simulink model "PV_UPQC_Final1_MAF_2018a (1)"  (R2018a)
settings: Solver=ode23tb  StartTime=0.0  StopTime=6  FixedStep=Ts_Power  RelTol=1e-4
PreLoadFcn:
  | Ts_Power=50e-6;
  | Ts_Control=100e-6;
InitFcn:
  | Ts_Power=50e-6;
  | Ts_Control=100e-6;
model workspace (MAT data in the model file):
  A = [0  0  0; -1  -1.5  -0.75; 0  1  0]
  B = [0.5; 0; 0]
  C = [0 -1.5 0]
  D = 0
  G = ss
  G.IOSize_ = [1 1]
  G.Data_ = ltipack.ssdata
  G.Data_.a = 0
  G.Data_.b = [0.5 0]
  G.Data_.c = [0.5; -0.5]
  G.Data_.d = [0  1; 0  0]
  G.Data_.Delay.Input = 0
  G.Data_.Delay.Output = 0
  G.Data_.Delay.Internal = 4
  G.Data_.Ts = 0
  Ga = ss
  Ga.IOSize_ = [1 1]
  Ga.Data_ = ltipack.ssdata
  Ga.Data_.a = [0  0  0; -1  -1.5  -0.75; 0  1  0]
  Ga.Data_.b = [0.5; 0; 0]
  Ga.Data_.c = [0 -1.5 0]
  Ga.Data_.d = 0
  Ga.Data_.Delay.Input = 0
  Ga.Data_.Delay.Output = 0
  Ga.Data_.Delay.Internal = []
  Ga.Data_.Ts = 0
  Gtf = tf
  Gtf.IOSize_ = [1 1]
  Gtf.Data_ = ltipack.tfdata
  Gtf.Data_.num = {[1 1.5 0.75 0]}
  Gtf.Data_.den = {[0 0 0.75 0]}
  Gtf.Data_.Delay.Input = 0
  Gtf.Data_.Delay.Output = 0
  Gtf.Data_.Delay.IO = 0
  Gtf.Data_.Ts = 0
  Ts = 2.5e-05
  s = tf
  s.IOSize_ = [1 1]
  s.Data_ = ltipack.tfdata
  s.Data_.num = {[1 0]}
  s.Data_.den = {[0 1]}
  s.Data_.Delay.Input = 0
  s.Data_.Delay.Output = 0
  s.Data_.Delay.IO = 0
  s.Data_.Ts = 0
libraries: powerlib x38, powerlib_meascontrol x12, simulink x4, dspstat3 x1, re_lib x1
Description:
  | Copyright 2008-2017 The MathWorks, Inc.
settings Model: Creator=MathWorks  LastModifiedBy=LMS Solution
settings SolverCC: SolverJacobianMethodControl=FullAnalytical  ZeroCrossAlgorithm=Adaptive  AlgebraicLoopSolver=LineSearch
settings DataIOCC: LimitDataPoints=on  SaveFormat=Array  SignalLoggingSaveFormat=ModelDataLogs
settings OptimizationCC: ExpressionDepthLimit=2147483647  LifeSpan=inf
settings DebuggingCC: UnderspecifiedInitializationDetection=Classic  MergeDetectMultiDrivingBlocksExec=none  SolverPrmCheckMsg=warning  FcnCallInpInsideContextMsg=warning  StateNameClashWarn=warning  SFUnexpectedBacktrackingDiag=warning  SFNoUnconditionalDefaultTransitionDiag=warning  SFExecutionAtInitializationDiag=none
settings HardwareCC: ProdBitPerPointer=32  ProdBitPerSizeT=32  ProdBitPerPtrDiffT=32  ProdLargestAtomicFloat=None  ProdIntDivRoundTo=Undefined  ProdEndianess=Unspecified  ProdWordSize=32  ProdHWDeviceType=32-bit Generic
settings ModelReferenceCC: PropagateSignalLabelsOutOfModel=off
settings CodeAppCC: StateflowObjectComments=on
settings GRTTargetCC: TargetLangStandard=C89/C90 (ANSI)  CombineOutputUpdateFcns=off  GRTInterface=on
settings ConfigComp: CovMetricSettings=dw  CovHtmlReporting=on  CovSaveCumulativeToWorkspaceVar=on  CovSaveSingleToWorkspaceVar=on  CovExternalEMLEnable=off  CovSFcnEnable=off
settings SimscapeCC: SimscapeNormalizeSystem=off

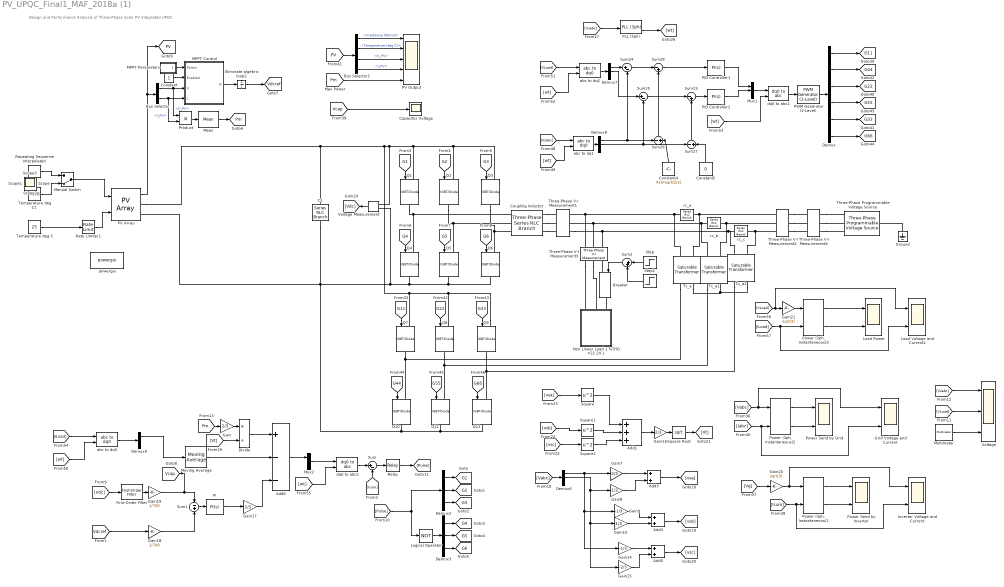
== system PV_UPQC_Final1_MAF_2018a (1) ==
  note: Design and Performance Analysis of Three-Phase Solar PV Integrated UPQC
  Add1 : Sum  Inputs=+++
  Add3 : Sum
  Add4 : Sum
  Add5 : Sum
  Add6 : Sum  Inputs=+--
  Breaker : powerlib/Elements/Breaker  InitialState=0  SwitchingTimes="[1/60  5/60]"  External=on  BreakerResistance=0.01  SnubberResistance=1e6  SnubberCapacitance=inf  Measurements=None  MoreParameters=on  NoBreakLoop=off
  Bus Selector : BusSelector  OutputSignals=V_PV,I_PV
  Bus Selector1 : BusSelector  OutputSignals=Irradiance (W/m2),Temperature (deg C),V_PV,I_PV
  C1 : powerlib/Elements/Series RLC Branch  LConnTagsString=__new0  RConnTagsString=__new0  BranchType=C  Resistance=1  Inductance=1e-3  SetiL0=off  InitialCurrent=0  Capacitance=6668e-6  Setx0=on  InitialVoltage=700  Measurements=None
  Capacitor Voltage : Scope
  Constant : Constant
  Constant4 : Constant  Value=415*sqrt(2/3)
  Constant5 : Constant  Value=0
  Coupling Inductor : powerlib/Elements/Three-Phase Series RLC Branch  LConnTagsString=A|B|C  RConnTagsString=A|B|C  BranchType=L  Resistance=0.09  Inductance=1.39e-3  Capacitance=1e-6  Measurements=None
  Demux : Demux  Outputs=6
  Demux{2..3,6..9} (6 alike) : Demux  Outputs=3
  Divide : Product  Inputs=*/
  Eliminate algebric loop2 : UnitDelay  InitialCondition=0.485  SampleTime=Ts_Control  HasFrameUpgradeWarning=on
  First-Order Filter : powerlib_meascontrol/Filters/First-Order Filter  FilterType=Lowpass  Tc=10e-3  Ts=0  Initialize=on  Vac_Init=[0, 0, 60]  Vdc_Init=0  PlotResponse=off  FreqRange="[0,  200,  1]"
  Gain : Gain  Gain=2/3
  Gain10 : Gain  Gain=1/3
  Gain14 : Gain  Gain=-1/3
  Gain15 : Gain  Gain=-2/3
  Gain16 : Gain  Gain=2/3
  Gain17 : Gain  Gain=1/3
  Gain18 : Gain  Gain=1/700
  Gain19 : Gain  Gain=1/700
  Gain20 : Gain  Gain=sqrt(3)
  Gain21 : Gain  Gain=sqrt(3)
  Gain7 : Gain  Gain=2/3
  Gain8 : Gain  Gain=1/3
  Gain9 : Gain  Gain=-1/3
  Grid Voltage and Current : Scope  NumInputPorts=2
  Ground : powerlib/Elements/Ground  LConnTagsString=a
  Inverter Voltage and Current : Scope  NumInputPorts=2
  Load Power : Scope  NumInputPorts=2
  Load Voltage and Current1 : Scope  NumInputPorts=2
  Logical Operator : Logic  Operator=NOT  IconShape=distinctive  AllPortsSameDT=off  OutDataTypeStr=boolean
  MPPT Parameters : Subsystem
  "MPPT Control  " : MATLAB Function  TreatAsAtomicUnit=on
  Manual Switch : ManualSwitch  CurrentSetting=0
  Mean : powerlib_meascontrol/Measurements/Mean  Freq=50  Vinit=0  Ts=0
  Moving Average : dspstat3/Moving Average  Method=Sliding window  ForgettingFactorPort=off  SpecifyWindowLength=on  WindowLength=4  ForgettingFactor=0.9  SimulateUsing=Code generation
  Multimeter : powerlib/Measurements/Multimeter  PhasorSimulation=off  OutputType=Complex  sel=[1 2 3]  L=3  Gain=[1 1 1]  yselected={'Ub: rc_a','Ub: rc_b','Ub: rc_c'};  PSBOutputType=1  PSBequivalent=0  AxesSetting=[0,0.1,-100,100]  Display=0  SavedBlockNames=-11
  Mux1 : Mux  Inputs=3
  Mux2 : Mux  Inputs=3
  "Non Linear Load { %THD =22.24 }" : Subsystem
      mask Display: fprintf('Non Linear\nLoad')
  PI : simulink/Continuous/PID Controller  Controller=PI  Form=Parallel  TimeDomain=Continuous-time  SampleTime=-1  IntegratorMethod=Forward Euler  FilterMethod=Forward Euler  ControllerParametersSource=internal  P=1000  I=1200  D=0  UseFilter=on  N=100  TunerSelectOption=Transfer Function Based (PID Tuner App)  InitialConditionSource=internal  InitialConditionForIntegrator=0  InitialConditionForFilter=0  DifferentiatorICPrevScaledInput=0  ExternalReset=none  TrackingMode=off  Kt=1  LimitOutput=off  UpperSaturationLimit=inf  LowerSaturationLimit=-inf  LinearizeAsGain=on  AntiWindupMode=none  Kb=1  POutMin=[]  POutMax=[]  IOutMin=[]  IOutMax=[]  DOutMin=[]  DOutMax=[]  NOutMin=[]  NOutMax=[]  SumOutMin=[]  SumOutMax=[]  SaturationOutMin=[]  SaturationOutMax=[]  PParamMin=[]  PParamMax=[]  IParamMin=[]  IParamMax=[]  DParamMin=[]  DParamMax=[]  NParamMin=[]  NParamMax=[]  KbParamMin=[]  KbParamMax=[]  KtParamMin=[]  KtParamMax=[]  KbOutMin=[]  KbOutMax=[]  KtOutMin=[]  KtOutMax=[]  IntegratorOutMin=[]  IntegratorOutMax=[]  FilterOutMin=[]  FilterOutMax=[]  SumI1OutMin=[]  SumI1OutMax=[]  SumI2OutMin=[]  SumI2OutMax=[]  SumI3OutMin=[]  SumI3OutMax=[]  SumDOutMin=[]  SumDOutMax=[]  DifferentiatorOutMin=[]  DifferentiatorOutMax=[]  FilterDiffOutCoefMin=[]  FilterDiffOutCoefMax=[]  ReciprocalOutMin=[]  ReciprocalOutMax=[]  SumDenOutMin=[]  SumDenOutMax=[]  SumNumOutMin=[]  SumNumOutMax=[]  DivideOutMin=[]  DivideOutMax=[]  IntegratorContinuousStateAttributes=''  IntegratorStateMustResolveToSignalObject=off  IntegratorRTWStateStorageClass=Auto  FilterContinuousStateAttributes=''  FilterStateMustResolveToSignalObject=off  FilterRTWStateStorageClass=Auto
  PID Controller1 : simulink/Continuous/PID Controller  Controller=PI  Form=Parallel  TimeDomain=Continuous-time  SampleTime=-1  IntegratorMethod=Forward Euler  FilterMethod=Forward Euler  ControllerParametersSource=internal  P=1  I=1  D=0  UseFilter=on  N=100  TunerSelectOption=Transfer Function Based (PID Tuner App)  InitialConditionSource=internal  InitialConditionForIntegrator=0  InitialConditionForFilter=0  DifferentiatorICPrevScaledInput=0  ExternalReset=none  TrackingMode=off  Kt=1  LimitOutput=off  UpperSaturationLimit=inf  LowerSaturationLimit=-inf  LinearizeAsGain=on  AntiWindupMode=none  Kb=1  POutMin=[]  POutMax=[]  IOutMin=[]  IOutMax=[]  DOutMin=[]  DOutMax=[]  NOutMin=[]  NOutMax=[]  SumOutMin=[]  SumOutMax=[]  SaturationOutMin=[]  SaturationOutMax=[]  PParamMin=[]  PParamMax=[]  IParamMin=[]  IParamMax=[]  DParamMin=[]  DParamMax=[]  NParamMin=[]  NParamMax=[]  KbParamMin=[]  KbParamMax=[]  KtParamMin=[]  KtParamMax=[]  KbOutMin=[]  KbOutMax=[]  KtOutMin=[]  KtOutMax=[]  IntegratorOutMin=[]  IntegratorOutMax=[]  FilterOutMin=[]  FilterOutMax=[]  SumI1OutMin=[]  SumI1OutMax=[]  SumI2OutMin=[]  SumI2OutMax=[]  SumI3OutMin=[]  SumI3OutMax=[]  SumDOutMin=[]  SumDOutMax=[]  DifferentiatorOutMin=[]  DifferentiatorOutMax=[]  FilterDiffOutCoefMin=[]  FilterDiffOutCoefMax=[]  ReciprocalOutMin=[]  ReciprocalOutMax=[]  SumDenOutMin=[]  SumDenOutMax=[]  SumNumOutMin=[]  SumNumOutMax=[]  DivideOutMin=[]  DivideOutMax=[]  IntegratorContinuousStateAttributes=''  IntegratorStateMustResolveToSignalObject=off  IntegratorRTWStateStorageClass=Auto  FilterContinuousStateAttributes=''  FilterStateMustResolveToSignalObject=off  FilterRTWStateStorageClass=Auto
  PID Controller2 : simulink/Continuous/PID Controller  Controller=PI  Form=Parallel  TimeDomain=Continuous-time  SampleTime=-1  IntegratorMethod=Forward Euler  FilterMethod=Forward Euler  ControllerParametersSource=internal  P=8  I=10  D=0  UseFilter=on  N=100  TunerSelectOption=Transfer Function Based (PID Tuner App)  InitialConditionSource=internal  InitialConditionForIntegrator=0  InitialConditionForFilter=0  DifferentiatorICPrevScaledInput=0  ExternalReset=none  TrackingMode=off  Kt=1  LimitOutput=off  UpperSaturationLimit=inf  LowerSaturationLimit=-inf  LinearizeAsGain=on  AntiWindupMode=none  Kb=1  POutMin=[]  POutMax=[]  IOutMin=[]  IOutMax=[]  DOutMin=[]  DOutMax=[]  NOutMin=[]  NOutMax=[]  SumOutMin=[]  SumOutMax=[]  SaturationOutMin=[]  SaturationOutMax=[]  PParamMin=[]  PParamMax=[]  IParamMin=[]  IParamMax=[]  DParamMin=[]  DParamMax=[]  NParamMin=[]  NParamMax=[]  KbParamMin=[]  KbParamMax=[]  KtParamMin=[]  KtParamMax=[]  KbOutMin=[]  KbOutMax=[]  KtOutMin=[]  KtOutMax=[]  IntegratorOutMin=[]  IntegratorOutMax=[]  FilterOutMin=[]  FilterOutMax=[]  SumI1OutMin=[]  SumI1OutMax=[]  SumI2OutMin=[]  SumI2OutMax=[]  SumI3OutMin=[]  SumI3OutMax=[]  SumDOutMin=[]  SumDOutMax=[]  DifferentiatorOutMin=[]  DifferentiatorOutMax=[]  FilterDiffOutCoefMin=[]  FilterDiffOutCoefMax=[]  ReciprocalOutMin=[]  ReciprocalOutMax=[]  SumDenOutMin=[]  SumDenOutMax=[]  SumNumOutMin=[]  SumNumOutMax=[]  DivideOutMin=[]  DivideOutMax=[]  IntegratorContinuousStateAttributes=''  IntegratorStateMustResolveToSignalObject=off  IntegratorRTWStateStorageClass=Auto  FilterContinuousStateAttributes=''  FilterStateMustResolveToSignalObject=off  FilterRTWStateStorageClass=Auto
  PLL (3ph) : powerlib_meascontrol/PLL/PLL (3ph)  Fmin=45  Par_Init=[0, 60]  ParK=[180, 3200, 1]  TcD=1e-4  MaxRateChangeFreq=12  FilterCutOffFreq=25  Ts=0  AGC=on
  PV Array : re_lib/Solar/PV Array  Npar=18  Nser=25  PlotType=array @ 25 deg.C & specified irradiances  S_vec="[ 1000  500  100 ]"  Temp_C_vec="[ 45 25  ]"  ModuleName=1Soltech 1STH-215-P  PlotWhenSelected=off  Pm=213.15  Ncell=60  Voc=36.3  Isc=7.84  Vm=29  Im=7.35  beta_Voc_pc=-0.36099  alpha_Isc_pc=0.102  beta_Voc=-0.13104  alpha_Isc=0.007997  IL=7.8649  I0=2.9259e-10  nI=0.98117  Rsh=313.3991  Rs=0.39383  RobustModel=off  RobustCellTemperature=25  BAL=on  Tc=1e-6  Tfilter=5e-5
  PV Output : Scope  NumInputPorts=5
  PWM Generator (2-Level) : powerlib_meascontrol/Pulse & Signal Generators/PWM Generator (2-Level)  ModulatorType=Three-phase bridge (6 pulses)  ModulatorMode=Unsynchronized  Fc=10e3  Pc=90  nF=27  MinMax="[ -1  1 ]"  SamplingTechnique=Natural  ModulatingSignals=off  m=0.8  Freq=60  Phase=0  Ts=0  ShowCarrierOutport=off
  "Power (3ph, Instantaneous)1" : powerlib_meascontrol/Measurements/Power (3ph, Instantaneous)
  "Power (3ph, Instantaneous)2" : powerlib_meascontrol/Measurements/Power (3ph, Instantaneous)
  "Power (3ph, Instantaneous)3" : powerlib_meascontrol/Measurements/Power (3ph, Instantaneous)
  Power Send by Grid : Scope  NumInputPorts=2
  Power Send by Inverter : Scope  NumInputPorts=2
  Product : Product
  Q{1..12} (12 alike) : powerlib/Power Electronics/IGBT//Diode  Ron=1e-3  Rs=1e5  Cs=inf  Measurements=off
  Rate Limiter1 : RateLimiter  RisingSlewLimit=100  FallingSlewLimit=-100  SampleTimeMode=inherited
  Relay : Relay  OnSwitchValue=0.1  OffSwitchValue=-0.1
  Repeating Sequence Interpolated : simulink/Sources/Repeating Sequence Interpolated  OutValues=[500 500 1000 1000 1000].'  TimeValues=[0 2 2.5 3 6].'  LookUpMeth=Interpolation-Use End Values  tsamp=0.01  OutMin=[]  OutMax=[]  OutDataTypeStr=double  OutputDataTypeScalingMode=double  OutDataType=fixdt(0,8)  OutScaling=2^-10
  Square : Math  Operator=square  SaturateOnIntegerOverflow=on
  Square Root : Sqrt  SaturateOnIntegerOverflow=on
  Square1 : Math  Operator=square  SaturateOnIntegerOverflow=on
  Square2 : Math  Operator=square  SaturateOnIntegerOverflow=on
  Step : Step  Before=1  After=0  SampleTime=0
  Step1 : Step  Time=1.2  SampleTime=0
  Sum : Sum  Inputs=|+-
  Sum1 : Sum  Inputs=-+
  Sum2 : Sum  Inputs=|++
  Sum23 : Sum  Inputs=|-+
  Sum24 : Sum  Inputs=|+-
  Sum25 : Sum  Inputs=|+-
  Sum26 : Sum  Inputs=-+
  Sum27 : Sum  Inputs=-+
  Sum28 : Sum  Inputs=|-+
  Tc_a : powerlib/Elements/Saturable Transformer  ThreeWindings=off  Hysteresis=off  DataFile='hysteresis.mat'  Measurements=None  UNITS=pu  NominalPower=[4000 50]  Winding1="[380  0.02  0.02 ]"  Winding2="[380  0.02  0.02]"  Winding3="[ 315e3  0.002  0.08 ]"  Saturation=[ 0 0 ;1.016 9.043]*1e-3  CoreLoss=[117 0]  BreakLoop=off  DiscreteSolver=Trapezoidal iterative  DataType=off  InitialFlux=0  TransfoNumber=1
      settings: SourceProductBaseCode=PS
  Tc_a1 : powerlib/Elements/Saturable Transformer  ThreeWindings=off  Hysteresis=off  DataFile='hysteresis.mat'  Measurements=None  UNITS=pu  NominalPower=[4000 50]  Winding1="[380  0.02  0.02 ]"  Winding2="[380  0.02  0.02]"  Winding3="[ 315e3  0.002  0.08 ]"  Saturation=[ 0 0 ;1.016 9.043]*1e-3  CoreLoss=[117 0]  BreakLoop=off  DiscreteSolver=Trapezoidal iterative  DataType=off  InitialFlux=0  TransfoNumber=1
      settings: SourceProductBaseCode=PS
  Tc_a2 : powerlib/Elements/Saturable Transformer  ThreeWindings=off  Hysteresis=off  DataFile='hysteresis.mat'  Measurements=None  UNITS=pu  NominalPower=[4000 50]  Winding1="[380  0.02  0.02 ]"  Winding2="[380  0.02  0.02]"  Winding3="[ 315e3  0.002  0.08 ]"  Saturation=[ 0 0 ;1.016 9.043]*1e-3  CoreLoss=[117 0]  BreakLoop=off  DiscreteSolver=Trapezoidal iterative  DataType=off  InitialFlux=0  TransfoNumber=1
      settings: SourceProductBaseCode=PS
  Temperature deg C : Constant  Value=25
  Temperature deg C1 : Constant  Value=1000
  Three-Phase Programmable Voltage Source : powerlib/Electrical Sources/Three-Phase Programmable Voltage Source  PositiveSequence=[400 0 50]  VariationEntity=Amplitude  VariationType=Table of time-amplitude pairs  VariationTypeAlt=Step  VariationStep=0.5  VariationRate=10  VariationMagnitude=0.3  VariationFrequency=2  VariationTiming=[1 2]  VariationPhaseA=off  Amplitudes=[1 0.8 1 1.2 1 1]  TimeValues=[0 3 3.5 4 4.5 5]  HarmonicGeneration=off  HarmonicA=[5 0.2 -25 0]  HarmonicB=[7 0.15 35 2]  Timing="[5  5.2]"  BusType=swing  Pref=0  Qref=0  Qmin=-inf  Qmax=inf
  Three-Phase V-I Measurement1 : powerlib/Measurements/Three-Phase V-I Measurement  VoltageMeasurement=phase-to-ground  SetLabelV=on  LabelV=Vg  Vpu=off  VpuLL=off  CurrentMeasurement=yes  SetLabelI=on  LabelI=Icom  Ipu=off  Pbase=100e6  Vbase=500e3  OutputType=Complex  PhasorSimulation=off  PSBequivalent=0
  Three-Phase V-I Measurement2 : powerlib/Measurements/Three-Phase V-I Measurement  VoltageMeasurement=phase-to-phase  SetLabelV=on  LabelV=Vabc  Vpu=off  VpuLL=off  CurrentMeasurement=yes  SetLabelI=on  LabelI=Iabc  Ipu=off  Pbase=100e6  Vbase=500e3  OutputType=Complex  PhasorSimulation=off  PSBequivalent=0
  Three-Phase V-I Measurement3 : powerlib/Measurements/Three-Phase V-I Measurement  VoltageMeasurement=phase-to-ground  SetLabelV=on  LabelV=VLoad  Vpu=off  VpuLL=off  CurrentMeasurement=yes  SetLabelI=on  LabelI=ILoad  Ipu=off  Pbase=100e6  Vbase=500e3  OutputType=Complex  PhasorSimulation=off  PSBequivalent=0
  Three-Phase V-I Measurement4 : powerlib/Measurements/Three-Phase V-I Measurement  VoltageMeasurement=phase-to-ground  SetLabelV=on  LabelV=Vsabc  Vpu=off  VpuLL=off  CurrentMeasurement=no  SetLabelI=on  LabelI=Iabc  Ipu=off  Pbase=100e6  Vbase=500e3  OutputType=Complex  PhasorSimulation=off  PSBequivalent=0
  Voltage : Scope  NumInputPorts=3
  Voltage Measurement : powerlib/Measurements/Voltage Measurement  PhasorSimulation=off  OutputType=Complex  PSBequivalent=0
  abc to dq1 : powerlib_meascontrol/Transformations/abc to dq0  Alignment=90 degrees behind phase A axis
  abc to dq2 : powerlib_meascontrol/Transformations/abc to dq0  Alignment=90 degrees behind phase A axis
  abc to dq3 : powerlib_meascontrol/Transformations/abc to dq0  Alignment=90 degrees behind phase A axis
  dq0 to abc1 : powerlib_meascontrol/Transformations/dq0 to abc  Alignment=90 degrees behind phase A axis
  dq0 to abc2 : powerlib_meascontrol/Transformations/dq0 to abc  Alignment=90 degrees behind phase A axis
  powergui : powerlib/powergui  Priority=1  SimulationMode=Discrete  SampleTime=1e-6  frequency=60  Iterations=50  frequencyindice=0  Pbase=100e6  ErrMax=1e-4  UnitsV=kV  UnitsW=MW  buscounter=0  FunctionMessages=off  echomessages=off  EnableUseOfTLC=off  CurrentSourceSwitches=off  DisableSnubberDevices=off  DisableRonSwitches=off  DisableVfSwitches=off  DisplayEquations=off  AutomaticDiscreteSolvers=off  SolverType=Tustin/Backward Euler (TBE)  Interpol=off  ExternalGateDelay=off  methode=off  Ts=100  x0status=blocks  SPID=on  SwTol=0  HookPort=off  NonlinearTolerance=1e-4  nMaxIteration=100  ContinueOnMaxIteration=off  RestoreLinks=warning  ResistiveCurrentMeasurement=off  Frange=[0:2:500]  Ylog=off  Xlog=on  ShowGrid=off  save=off  variable=ZData  structure=ScopeData5  ZoomFFT=on  StartTime=0.2  cycles=1  DisplayStyle=1  fundamental=50  FreqAxis=off  MaxFrequency=2500  frequencyindicesteady=1  RmsSteady=1  display=off
  rc_a : powerlib/Elements/Series RLC Branch  LConnTagsString=__new0  RConnTagsString=__new0  BranchType=RC  Resistance=1  Inductance=1e-3  SetiL0=off  InitialCurrent=0  Capacitance=100e-6  Setx0=off  InitialVoltage=0  Measurements=Branch voltage
  rc_b : powerlib/Elements/Series RLC Branch  LConnTagsString=__new0  RConnTagsString=__new0  BranchType=RC  Resistance=1  Inductance=1e-3  SetiL0=off  InitialCurrent=0  Capacitance=100e-6  Setx0=off  InitialVoltage=0  Measurements=Branch voltage
  rc_c : powerlib/Elements/Series RLC Branch  LConnTagsString=__new0  RConnTagsString=__new0  BranchType=RC  Resistance=1  Inductance=1e-3  SetiL0=off  InitialCurrent=0  Capacitance=100e-6  Setx0=off  InitialVoltage=0  Measurements=Branch voltage
  Scope{,1..3} (4 alike) : Scope
  tag scope: G11=global, G1=global, G22=global, G2=global, G33=global, G3=global, G44=global, G4=global, G55=global, G5=global, G66=global, G6=global, PV=global, Pm=global, Vcap=global, Vdcref=global
  wires:
  PV Array/1 -> [PV], Bus Selector/1
  Bus Selector/2 -> Product/2, "MPPT Control  "/4(I)  "<I_PV>"
  MPPT Parameters/1(Param) -> "MPPT Control  "/1(Param)
  Constant/1 -> "MPPT Control  "/2(Enabled)
  Bus Selector/1 -> Product/1, "MPPT Control  "/3(V)  "<V_PV>"
  "MPPT Control  "/1(D) -> Eliminate algebric loop2/1
  Product/1 -> Mean/1
  [G5] -> Q5/1
  [G4] -> Q4/1
  Demux2/2 -> [G2]
  Demux3/2 -> [G5]
  [G1] -> Q1/1
  Demux3/1 -> [G4]
  Demux2/3 -> [G3]
  Demux2/1 -> [G1]
  [G3] -> Q3/1
  [G2] -> Q2/1
  Logical Operator/1 -> Demux3/1
  [G6] -> Q6/1
  Demux3/3 -> [G6]
  Mean/1 -> [Pm]
  [Pulse] -> Logical Operator/1, Demux2/1
  [Vdcref] -> Gain18/1
  Relay/1 -> [Pulse]
  Sum/1 -> Relay/1
  [Icom] -> Sum/2
  Gain/1 -> Divide/1
  Sum1/1 -> PI/1
  Voltage Measurement/1 -> [Vdc]
  [Vdc] -> First-Order Filter/1
  First-Order Filter/1 -> Gain19/1
  Eliminate algebric loop2/1 -> [Vdcref]
  [Pm] -> Gain/1
  Add3/1 -> [vsa]
  Gain7/1 -> Add3/1
  Gain8/1 -> Add3/2
  [Vabc] -> Demux6/1
  Gain9/1 -> Add4/1
  Gain10/1 -> Add4/2
  Add4/1 -> [vsb]
  Add5/1 -> [vsc]
  Demux6/1 -> Gain14/1, Gain9/1, Gain7/1
  Demux6/2 -> Gain15/1, Gain10/1, Gain8/1
  Gain15/1 -> Add5/2
  Gain14/1 -> Add5/1
  Add1/1 -> Gain16/1
  Square2/1 -> Add1/3
  Square/1 -> Add1/1
  [vsa] -> Square/1
  Square Root/1 -> [Vt]
  Gain16/1 -> Square Root/1
  Square1/1 -> Add1/2
  [vsb] -> Square1/1
  [vsc] -> Square2/1
  [Vt] -> Divide/2
  PI/1 -> Gain17/1
  Gain18/1 -> Sum1/2
  Gain19/1 -> Sum1/1, [Vcap]
  "Power (3ph, Instantaneous)2"/1 -> Power Send by Grid/1
  "Power (3ph, Instantaneous)1"/2 -> Power Send by Inverter/2
  [Vabc] -> Grid Voltage and Current/1, "Power (3ph, Instantaneous)2"/1
  [Iabc] -> Grid Voltage and Current/2, "Power (3ph, Instantaneous)2"/2
  "Power (3ph, Instantaneous)2"/2 -> Power Send by Grid/2
  [Vg] -> Gain20/1
  [Vcap] -> Capacitor Voltage/1
  [PV] -> Bus Selector1/1
  "Power (3ph, Instantaneous)1"/1 -> Power Send by Inverter/1
  [Pm] -> PV Output/5
  Bus Selector1/1 -> PV Output/1  "<Irradiance (W/m2)>"
  [Icom] -> Inverter Voltage and Current/2, "Power (3ph, Instantaneous)1"/2
  Bus Selector1/3 -> PV Output/3  "<V_PV>"
  Bus Selector1/2 -> PV Output/2  "<Temperature (deg C)>"
  Bus Selector1/4 -> PV Output/4  "<I_PV>"
  Divide/1 -> Add6/1
  Gain17/1 -> Add6/3
  [G33] -> Q9/1
  [G11] -> Q7/1
  [G22] -> Q8/1
  [G66] -> Q12/1
  [G44] -> Q10/1
  [G55] -> Q11/1
  Temperature deg C/1 -> Rate Limiter1/1
  Manual Switch/1 -> PV Array/1
  Rate Limiter1/1 -> PV Array/2
  Demux8/2 -> Sum27/1, Sum25/2
  Demux8/1 -> Sum26/1, Sum24/2
  Constant4/1 -> Sum26/2
  Constant5/1 -> Sum27/2
  Sum27/1 -> Sum23/2
  Sum26/1 -> Sum28/2
  [Vsabc] -> abc to dq1/1
  Sum24/1 -> Sum28/1
  Sum23/1 -> PID Controller2/1
  Demux7/2 -> Sum25/1
  [wt] -> abc to dq1/2
  Sum28/1 -> PID Controller1/1
  abc to dq1/1 -> Demux8/1
  [wt] -> dq0 to abc1/2
  abc to dq2/1 -> Demux7/1
  [VLoad] -> abc to dq2/1
  Demux7/1 -> Sum24/1
  [Vsabc] -> PLL (3ph)/1
  Mux1/1 -> dq0 to abc1/1
  [wt] -> abc to dq2/2
  PLL (3ph)/2 -> [wt]
  PID Controller1/1 -> Mux1/1
  Sum25/1 -> Sum23/1
  PID Controller2/1 -> Mux1/2
  dq0 to abc1/1 -> PWM Generator (2-Level)/1
  PWM Generator (2-Level)/1 -> Demux/1
  Demux/1 -> [G11]
  [ILoad] -> abc to dq3/1
  [wt] -> abc to dq3/2
  abc to dq3/1 -> Demux9/1
  Demux9/1 -> Moving Average/1
  Mux2/1 -> dq0 to abc2/1
  Add6/1 -> Mux2/1
  [wt] -> dq0 to abc2/2
  dq0 to abc2/1 -> Sum/1
  Gain20/1 -> Inverter Voltage and Current/1, "Power (3ph, Instantaneous)1"/1
  [VLoad] -> Load Voltage and Current1/1, Gain21/1
  [ILoad] -> Load Voltage and Current1/2, "Power (3ph, Instantaneous)3"/2
  Gain21/1 -> "Power (3ph, Instantaneous)3"/1
  "Power (3ph, Instantaneous)3"/1 -> Load Power/1
  "Power (3ph, Instantaneous)3"/2 -> Load Power/2
  Demux/2 -> [G44]
  Demux/3 -> [G22]
  Demux/4 -> [G55]
  Demux/5 -> [G33]
  Demux/6 -> [G66]
  Multimeter/1 -> Voltage/3
  [VLoad] -> Voltage/2
  [Vsabc] -> Voltage/1
  Sum2/1 -> Breaker/1
  Temperature deg C1/1 -> Manual Switch/2
  Repeating Sequence Interpolated/1 -> Manual Switch/1
  Step/1 -> Sum2/1
  Step1/1 -> Sum2/2
  Moving Average/1 -> Add6/2
  connections:
  Q11/RConn1 -- PV Array/RConn2 -- C1/RConn1 -- Q6/RConn1 -- Q5/RConn1 -- Q4/RConn1 -- Voltage Measurement/LConn2 -- Q10/RConn1 -- Q12/RConn1
  Q9/LConn1 -- Q8/LConn1 -- PV Array/RConn1 -- C1/LConn1 -- Voltage Measurement/LConn1 -- Q1/LConn1 -- Q2/LConn1 -- Q3/LConn1 -- Q7/LConn1
  Q3/RConn1 -- Coupling Inductor/LConn3 -- Q6/LConn1
  Q4/LConn1 -- Q1/RConn1 -- Coupling Inductor/LConn1
  Q5/LConn1 -- Q2/RConn1 -- Coupling Inductor/LConn2
  Coupling Inductor/RConn3 -- Three-Phase V-I Measurement1/LConn3
  Coupling Inductor/RConn1 -- Three-Phase V-I Measurement1/LConn1
  Coupling Inductor/RConn2 -- Three-Phase V-I Measurement1/LConn2
  Ground/LConn1 -- Three-Phase Programmable Voltage Source/LConn1
  Tc_a2/RConn2 -- Three-Phase V-I Measurement2/RConn3 -- rc_c/LConn1
  Tc_a/RConn1 -- rc_a/RConn1 -- Three-Phase V-I Measurement1/RConn1 -- Three-Phase V-I Measurement3/LConn1
  rc_c/RConn1 -- Three-Phase V-I Measurement3/LConn3 -- Three-Phase V-I Measurement1/RConn3 -- Tc_a2/RConn1
  Tc_a1/RConn2 -- Three-Phase V-I Measurement2/RConn2 -- rc_b/LConn1
  Tc_a1/RConn1 -- rc_b/RConn1 -- Three-Phase V-I Measurement3/LConn2 -- Three-Phase V-I Measurement1/RConn2
  Tc_a/RConn2 -- Three-Phase V-I Measurement2/RConn1 -- rc_a/LConn1
  Q7/RConn1 -- Tc_a/LConn1 -- Q10/LConn1
  Q8/RConn1 -- Tc_a1/LConn1 -- Q11/LConn1
  Q9/RConn1 -- Tc_a2/LConn1 -- Q12/LConn1
  Tc_a/LConn2 -- Tc_a2/LConn2 -- Tc_a1/LConn2
  Three-Phase V-I Measurement3/RConn1 -- "Non Linear Load { %THD =22.24 }"/LConn1
  Three-Phase V-I Measurement3/RConn2 -- "Non Linear Load { %THD =22.24 }"/LConn2
  Breaker/LConn1 -- Three-Phase V-I Measurement3/RConn3
  Breaker/RConn1 -- "Non Linear Load { %THD =22.24 }"/LConn3
  Three-Phase V-I Measurement4/RConn1 -- Three-Phase Programmable Voltage Source/RConn1
  Three-Phase V-I Measurement4/RConn2 -- Three-Phase Programmable Voltage Source/RConn2
  Three-Phase V-I Measurement4/RConn3 -- Three-Phase Programmable Voltage Source/RConn3
  Three-Phase V-I Measurement2/LConn1 -- Three-Phase V-I Measurement4/LConn1
  Three-Phase V-I Measurement2/LConn2 -- Three-Phase V-I Measurement4/LConn2
  Three-Phase V-I Measurement2/LConn3 -- Three-Phase V-I Measurement4/LConn3

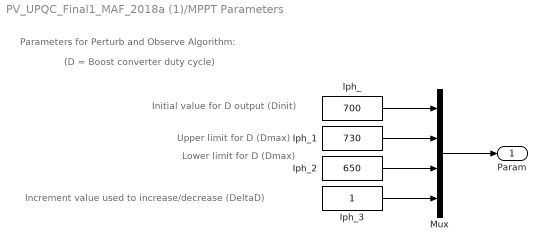
== system PV_UPQC_Final1_MAF_2018a (1)/MPPT Parameters ==
  note: Upper limit for D (Dmax)
  note: Increment value used to increase/decrease (DeltaD)
  note: Initial value for D output (Dinit)
  note: (D = Boost converter duty cycle)
  note: Lower limit for D (Dmax)
  note: Parameters for Perturb and Observe Algorithm:
  Iph_ : Constant  Value=700
  Iph_1 : Constant  Value=730
  Iph_2 : Constant  Value=650
  Iph_3 : Constant
  Mux : Mux
  Param : Outport
  wires:
  Iph_/1 -> Mux/1
  Iph_1/1 -> Mux/2
  Iph_2/1 -> Mux/3
  Iph_3/1 -> Mux/4
  Mux/1 -> Param/1

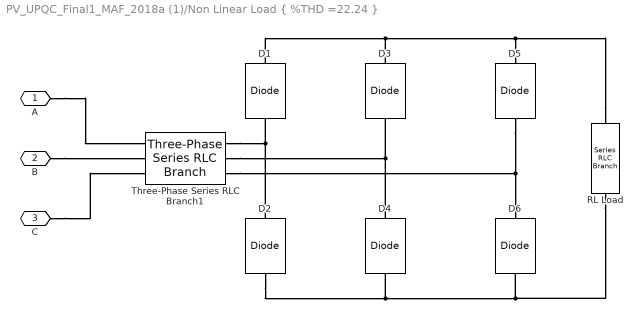
== system PV_UPQC_Final1_MAF_2018a (1)/Non Linear Load { %THD =22.24 } ==
  D{1..6} (6 alike) : powerlib/Power Electronics/Diode  Ron=0.001  Lon=0  Vf=0.8  IC=0  UseSnubber=off  Rs=500  Cs=250e-9  Measurements=off
  RL Load : powerlib/Elements/Series RLC Branch  LConnTagsString=__new0  RConnTagsString=__new0  BranchType=RL  Resistance=30  Inductance=0.15e-3  SetiL0=off  InitialCurrent=0  Capacitance=1e-6  Setx0=off  InitialVoltage=0  Measurements=None
  Three-Phase Series RLC Branch1 : powerlib/Elements/Three-Phase Series RLC Branch  LConnTagsString=A|B|C  RConnTagsString=A|B|C  BranchType=RL  Resistance=0.4  Inductance=15e-3  Capacitance=1e-6  Measurements=None
  A : PMIOPort  Side=Left
  B : PMIOPort  Port=2  Side=Left
  C : PMIOPort  Port=3  Side=Left
  connections:
  C/RConn1 -- Three-Phase Series RLC Branch1/LConn3
  B/RConn1 -- Three-Phase Series RLC Branch1/LConn2
  A/RConn1 -- Three-Phase Series RLC Branch1/LConn1
  Three-Phase Series RLC Branch1/RConn3 -- D6/RConn1 -- D5/LConn1
  Three-Phase Series RLC Branch1/RConn2 -- D4/RConn1 -- D3/LConn1
  RL Load/RConn1 -- D6/LConn1 -- D4/LConn1 -- D2/LConn1
  RL Load/LConn1 -- D5/RConn1 -- D3/RConn1 -- D1/RConn1
  Three-Phase Series RLC Branch1/RConn1 -- D2/RConn1 -- D1/LConn1

== matlab function PV_UPQC_Final1_MAF_2018a (1)/MPPT Control   ==
  settings: updateMethod=DISCRETE  sampleTime=Ts_Control
  data: Param input; Enabled input; V input =V; I input; D output
function D  = PandO(Param, Enabled, V, I)

% MPPT controller based on the Perturb & Observe algorithm.

% D output = Duty cycle of the boost converter (value between 0 and 1)
%
% Enabled input = 1 to enable the MPPT controller
% V input = PV array terminal voltage (V)
% I input = PV array current (A)
%
% Param input:
Dinit = Param(1);  %Initial value for D output
Dmax = Param(2);   %Maximum value for D
Dmin = Param(3);   %Minimum value for D
deltaD = Param(4); %Increment value used to increase/decrease the duty cycle D
% ( increasing D = decreasing Vref )
%  

persistent Vold Pold Dold;

dataType = 'double';

if isempty(Vold)
    Vold=0;
    Pold=0;
    Dold=Dinit;
end
P= V*I;
dV= V - Vold;
dP= P - Pold;

if dP ~= 0 & Enabled ~=0
    if dP < 0
        if dV < 0
            D = Dold - deltaD;
        else
            D = Dold + deltaD;
        end
    else
        if dV < 0
            D = Dold + deltaD;
        else
            D = Dold - deltaD;
        end    
    end
else D=Dold;
end

if D >= Dmax | D<= Dmin
    D=Dold;
end

Dold=D;
Vold=V;
Pold=P;
